simulink model "analiseLongitudinal"  (R2016a)
settings: Solver=ode4  StartTime=0.0  StopTime=60  FixedStep=0.01  RelTol=1e-3
undefined symbols (not defined in the file): aeronave, Ch, Ctheta, CVt, degtorad, Kh, Kq, Ktheta, KVt
libraries: simulink x9, cstblocks x4
settings Model: PauseTimes=20  Creator=IEE  LastModifiedBy=Pegasus
settings DataIOCC: LimitDataPoints=on  SaveFormat=Array
settings DebuggingCC: UnderspecifiedInitializationDetection=Classic  MergeDetectMultiDrivingBlocksExec=none  SolverPrmCheckMsg=warning  StateNameClashWarn=warning
settings HardwareCC: ProdBitPerPointer=32  ProdLargestAtomicFloat=None  ProdIntDivRoundTo=Undefined  ProdEndianess=Unspecified  ProdWordSize=32  ProdHWDeviceType=32-bit Generic
settings ModelReferenceCC: PropagateSignalLabelsOutOfModel=off
settings ConfigComp: CovModelRefEnable=Off

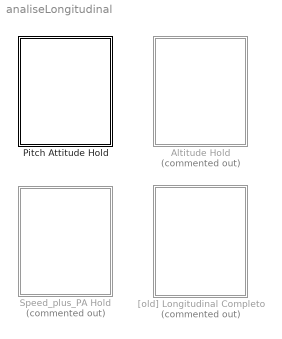
== system analiseLongitudinal ==
  Altitude Hold : Subsystem  Commented=on
  Pitch Attitude Hold : Subsystem
  Speed_plus_PA Hold : Subsystem  Commented=on
  "[old] Longitudinal Completo" : Subsystem  Commented=on

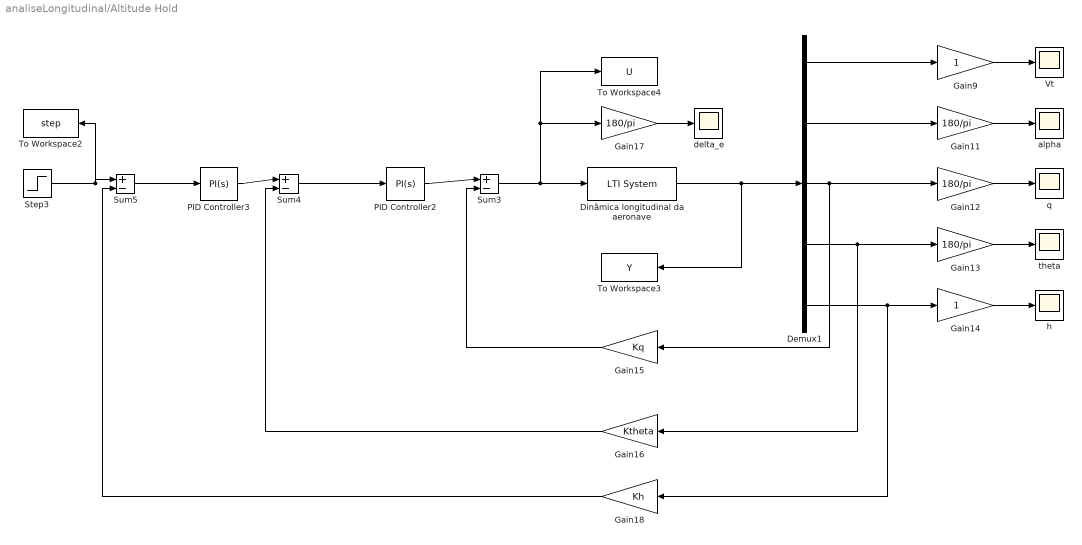
== system analiseLongitudinal/Altitude Hold ==
  Demux1 : Demux  Outputs=5
  Dinâmica longitudinal da aeronave : cstblocks/LTI System  sys=aeronave(:,2)  IC=[]
  Gain{11..13,17} (4 alike) : Gain  Gain=180/pi
  Gain14 : Gain
  Gain15 : Gain  Gain=Kq
  Gain16 : Gain  Gain=Ktheta
  Gain18 : Gain  Gain=Kh
  Gain9 : Gain
  PID Controller2 : simulink/Continuous/PID Controller  Controller=PI  TimeDomain=Continuous-time  SampleTime=-1  IntegratorMethod=Forward Euler  FilterMethod=Forward Euler  Form=Parallel  UseFilter=on  ControllerParametersSource=internal  P=Ctheta.Kp  I=Ctheta.Ki  D=0  N=100  InitialConditionSource=internal  InitialConditionForIntegrator=0  InitialConditionForFilter=0  ExternalReset=none  LimitOutput=off  UpperSaturationLimit=inf  LowerSaturationLimit=-inf  LinearizeAsGain=on  AntiWindupMode=none  Kb=1  TrackingMode=off  Kt=1  PParamMin=[]  PParamMax=[]  IParamMin=[]  IParamMax=[]  DParamMin=[]  DParamMax=[]  NParamMin=[]  NParamMax=[]  KbParamMin=[]  KbParamMax=[]  KtParamMin=[]  KtParamMax=[]  POutMin=[]  POutMax=[]  IOutMin=[]  IOutMax=[]  DOutMin=[]  DOutMax=[]  NOutMin=[]  NOutMax=[]  KbOutMin=[]  KbOutMax=[]  KtOutMin=[]  KtOutMax=[]  IntegratorOutMin=[]  IntegratorOutMax=[]  FilterOutMin=[]  FilterOutMax=[]  SumOutMin=[]  SumOutMax=[]  SumI1OutMin=[]  SumI1OutMax=[]  SumI2OutMin=[]  SumI2OutMax=[]  SumI3OutMin=[]  SumI3OutMax=[]  SumDOutMin=[]  SumDOutMax=[]  SaturationOutMin=[]  SaturationOutMax=[]  IntegratorContinuousStateAttributes=''  IntegratorStateMustResolveToSignalObject=off  IntegratorRTWStateStorageClass=Auto  FilterContinuousStateAttributes=''  FilterStateMustResolveToSignalObject=off  FilterRTWStateStorageClass=Auto  DifferentiatorICPrevScaledInput=0  DifferentiatorOutMin=[]  DifferentiatorOutMax=[]
  PID Controller3 : simulink/Continuous/PID Controller  Controller=PI  TimeDomain=Continuous-time  SampleTime=-1  IntegratorMethod=Forward Euler  FilterMethod=Forward Euler  Form=Parallel  UseFilter=on  ControllerParametersSource=internal  P=Ch.Kp  I=Ch.Ki  D=0  N=100  InitialConditionSource=internal  InitialConditionForIntegrator=0  InitialConditionForFilter=0  ExternalReset=none  LimitOutput=off  UpperSaturationLimit=inf  LowerSaturationLimit=-inf  LinearizeAsGain=on  AntiWindupMode=none  Kb=1  TrackingMode=off  Kt=1  PParamMin=[]  PParamMax=[]  IParamMin=[]  IParamMax=[]  DParamMin=[]  DParamMax=[]  NParamMin=[]  NParamMax=[]  KbParamMin=[]  KbParamMax=[]  KtParamMin=[]  KtParamMax=[]  POutMin=[]  POutMax=[]  IOutMin=[]  IOutMax=[]  DOutMin=[]  DOutMax=[]  NOutMin=[]  NOutMax=[]  KbOutMin=[]  KbOutMax=[]  KtOutMin=[]  KtOutMax=[]  IntegratorOutMin=[]  IntegratorOutMax=[]  FilterOutMin=[]  FilterOutMax=[]  SumOutMin=[]  SumOutMax=[]  SumI1OutMin=[]  SumI1OutMax=[]  SumI2OutMin=[]  SumI2OutMax=[]  SumI3OutMin=[]  SumI3OutMax=[]  SumDOutMin=[]  SumDOutMax=[]  SaturationOutMin=[]  SaturationOutMax=[]  IntegratorContinuousStateAttributes=''  IntegratorStateMustResolveToSignalObject=off  IntegratorRTWStateStorageClass=Auto  FilterContinuousStateAttributes=''  FilterStateMustResolveToSignalObject=off  FilterRTWStateStorageClass=Auto  DifferentiatorICPrevScaledInput=0  DifferentiatorOutMin=[]  DifferentiatorOutMax=[]
  Step3 : Step  Time=20  After=5  SampleTime=0
  Sum3 : Sum  Inputs=|+-
  Sum4 : Sum  Inputs=|+-
  Sum5 : Sum  Inputs=|+-
  To Workspace2 : ToWorkspace  VariableName=step  SaveFormat=Timeseries  SampleTime=-1
  To Workspace3 : ToWorkspace  VariableName=Y  SaveFormat=Timeseries  SampleTime=-1
  To Workspace4 : ToWorkspace  VariableName=U  SaveFormat=Timeseries  SampleTime=-1
  Vt : Scope
  alpha : Scope
  delta_e : Scope
  h : Scope
  q : Scope
  theta : Scope
  wires:
  Demux1/1 -> Gain9/1
  Gain12/1 -> q/1
  Gain14/1 -> h/1
  Gain13/1 -> theta/1
  Demux1/2 -> Gain11/1
  Demux1/3 -> Gain15/1, Gain12/1
  Gain9/1 -> Vt/1
  Gain15/1 -> Sum3/2
  Gain11/1 -> alpha/1
  Gain16/1 -> Sum4/2
  PID Controller2/1 -> Sum3/1
  Gain17/1 -> delta_e/1
  Demux1/4 -> Gain16/1, Gain13/1
  Dinâmica longitudinal da aeronave/1 -> To Workspace3/1, Demux1/1
  Sum3/1 -> To Workspace4/1, Gain17/1, Dinâmica longitudinal da aeronave/1
  Demux1/5 -> Gain18/1, Gain14/1
  Step3/1 -> To Workspace2/1, Sum5/1
  Gain18/1 -> Sum5/2
  Sum5/1 -> PID Controller3/1
  PID Controller3/1 -> Sum4/1
  Sum4/1 -> PID Controller2/1

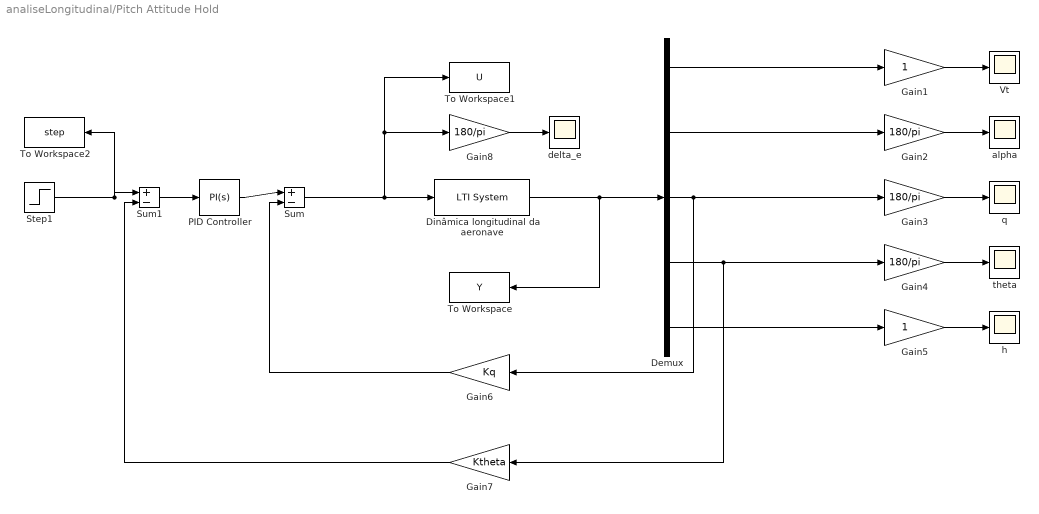
== system analiseLongitudinal/Pitch Attitude Hold ==
  Demux : Demux  Outputs=5
  Dinâmica longitudinal da aeronave : cstblocks/LTI System  sys=aeronave(:,2)  IC=[]
  Gain1 : Gain
  Gain{2..4,8} (4 alike) : Gain  Gain=180/pi
  Gain5 : Gain
  Gain6 : Gain  Gain=Kq
  Gain7 : Gain  Gain=Ktheta
  PID Controller : simulink/Continuous/PID Controller  Controller=PI  TimeDomain=Continuous-time  SampleTime=-1  IntegratorMethod=Forward Euler  FilterMethod=Forward Euler  Form=Parallel  UseFilter=on  ControllerParametersSource=internal  P=Ctheta.Kp  I=Ctheta.Ki  D=0  N=100  InitialConditionSource=internal  InitialConditionForIntegrator=0  InitialConditionForFilter=0  ExternalReset=none  LimitOutput=off  UpperSaturationLimit=inf  LowerSaturationLimit=-inf  LinearizeAsGain=on  AntiWindupMode=none  Kb=1  TrackingMode=off  Kt=1  PParamMin=[]  PParamMax=[]  IParamMin=[]  IParamMax=[]  DParamMin=[]  DParamMax=[]  NParamMin=[]  NParamMax=[]  KbParamMin=[]  KbParamMax=[]  KtParamMin=[]  KtParamMax=[]  POutMin=[]  POutMax=[]  IOutMin=[]  IOutMax=[]  DOutMin=[]  DOutMax=[]  NOutMin=[]  NOutMax=[]  KbOutMin=[]  KbOutMax=[]  KtOutMin=[]  KtOutMax=[]  IntegratorOutMin=[]  IntegratorOutMax=[]  FilterOutMin=[]  FilterOutMax=[]  SumOutMin=[]  SumOutMax=[]  SumI1OutMin=[]  SumI1OutMax=[]  SumI2OutMin=[]  SumI2OutMax=[]  SumI3OutMin=[]  SumI3OutMax=[]  SumDOutMin=[]  SumDOutMax=[]  SaturationOutMin=[]  SaturationOutMax=[]  IntegratorContinuousStateAttributes=''  IntegratorStateMustResolveToSignalObject=off  IntegratorRTWStateStorageClass=Auto  FilterContinuousStateAttributes=''  FilterStateMustResolveToSignalObject=off  FilterRTWStateStorageClass=Auto  DifferentiatorICPrevScaledInput=0  DifferentiatorOutMin=[]  DifferentiatorOutMax=[]
  Step1 : Step  Time=20  After=degtorad(5)  SampleTime=0
  Sum : Sum  Inputs=|+-
  Sum1 : Sum  Inputs=|+-
  To Workspace : ToWorkspace  VariableName=Y  SaveFormat=Timeseries  SampleTime=-1
  To Workspace1 : ToWorkspace  VariableName=U  SaveFormat=Timeseries  SampleTime=-1
  To Workspace2 : ToWorkspace  VariableName=step  SaveFormat=Timeseries  SampleTime=-1
  Vt : Scope
  alpha : Scope
  delta_e : Scope
  h : Scope
  q : Scope
  theta : Scope
  wires:
  Demux/1 -> Gain1/1
  Gain3/1 -> q/1
  Gain5/1 -> h/1
  Demux/5 -> Gain5/1
  Gain4/1 -> theta/1
  Demux/2 -> Gain2/1
  Demux/3 -> Gain6/1, Gain3/1
  Gain1/1 -> Vt/1
  Gain6/1 -> Sum/2
  Gain2/1 -> alpha/1
  Gain7/1 -> Sum1/2
  PID Controller/1 -> Sum/1
  Sum1/1 -> PID Controller/1
  Step1/1 -> To Workspace2/1, Sum1/1
  Gain8/1 -> delta_e/1
  Demux/4 -> Gain7/1, Gain4/1
  Dinâmica longitudinal da aeronave/1 -> To Workspace/1, Demux/1
  Sum/1 -> To Workspace1/1, Gain8/1, Dinâmica longitudinal da aeronave/1

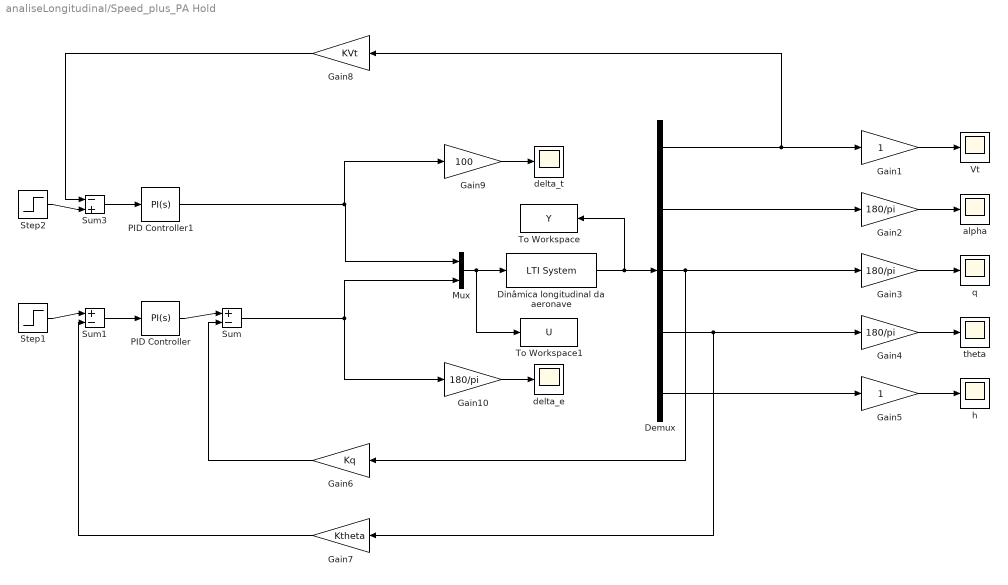
== system analiseLongitudinal/Speed_plus_PA Hold ==
  Demux : Demux  Outputs=5
  Dinâmica longitudinal da aeronave : cstblocks/LTI System  sys=aeronave  IC=[]
  Gain1 : Gain
  Gain{2..4,10} (4 alike) : Gain  Gain=180/pi
  Gain5 : Gain
  Gain6 : Gain  Gain=Kq
  Gain7 : Gain  Gain=Ktheta
  Gain8 : Gain  Gain=KVt
  Gain9 : Gain  Gain=100
  Mux : Mux  Inputs=2
  PID Controller : simulink/Continuous/PID Controller  Controller=PI  TimeDomain=Continuous-time  SampleTime=-1  IntegratorMethod=Forward Euler  FilterMethod=Forward Euler  Form=Parallel  UseFilter=on  ControllerParametersSource=internal  P=Ctheta.Kp  I=Ctheta.Ki  D=0  N=100  InitialConditionSource=internal  InitialConditionForIntegrator=0  InitialConditionForFilter=0  ExternalReset=none  LimitOutput=off  UpperSaturationLimit=inf  LowerSaturationLimit=-inf  LinearizeAsGain=on  AntiWindupMode=none  Kb=1  TrackingMode=off  Kt=1  PParamMin=[]  PParamMax=[]  IParamMin=[]  IParamMax=[]  DParamMin=[]  DParamMax=[]  NParamMin=[]  NParamMax=[]  KbParamMin=[]  KbParamMax=[]  KtParamMin=[]  KtParamMax=[]  POutMin=[]  POutMax=[]  IOutMin=[]  IOutMax=[]  DOutMin=[]  DOutMax=[]  NOutMin=[]  NOutMax=[]  KbOutMin=[]  KbOutMax=[]  KtOutMin=[]  KtOutMax=[]  IntegratorOutMin=[]  IntegratorOutMax=[]  FilterOutMin=[]  FilterOutMax=[]  SumOutMin=[]  SumOutMax=[]  SumI1OutMin=[]  SumI1OutMax=[]  SumI2OutMin=[]  SumI2OutMax=[]  SumI3OutMin=[]  SumI3OutMax=[]  SumDOutMin=[]  SumDOutMax=[]  SaturationOutMin=[]  SaturationOutMax=[]  IntegratorContinuousStateAttributes=''  IntegratorStateMustResolveToSignalObject=off  IntegratorRTWStateStorageClass=Auto  FilterContinuousStateAttributes=''  FilterStateMustResolveToSignalObject=off  FilterRTWStateStorageClass=Auto  DifferentiatorICPrevScaledInput=0  DifferentiatorOutMin=[]  DifferentiatorOutMax=[]
  PID Controller1 : simulink/Continuous/PID Controller  Controller=PI  TimeDomain=Continuous-time  SampleTime=-1  IntegratorMethod=Forward Euler  FilterMethod=Forward Euler  Form=Parallel  UseFilter=on  ControllerParametersSource=internal  P=CVt.Kp  I=CVt.Ki  D=0  N=100  InitialConditionSource=internal  InitialConditionForIntegrator=0  InitialConditionForFilter=0  ExternalReset=none  LimitOutput=off  UpperSaturationLimit=inf  LowerSaturationLimit=-inf  LinearizeAsGain=on  AntiWindupMode=none  Kb=1  TrackingMode=off  Kt=1  PParamMin=[]  PParamMax=[]  IParamMin=[]  IParamMax=[]  DParamMin=[]  DParamMax=[]  NParamMin=[]  NParamMax=[]  KbParamMin=[]  KbParamMax=[]  KtParamMin=[]  KtParamMax=[]  POutMin=[]  POutMax=[]  IOutMin=[]  IOutMax=[]  DOutMin=[]  DOutMax=[]  NOutMin=[]  NOutMax=[]  KbOutMin=[]  KbOutMax=[]  KtOutMin=[]  KtOutMax=[]  IntegratorOutMin=[]  IntegratorOutMax=[]  FilterOutMin=[]  FilterOutMax=[]  SumOutMin=[]  SumOutMax=[]  SumI1OutMin=[]  SumI1OutMax=[]  SumI2OutMin=[]  SumI2OutMax=[]  SumI3OutMin=[]  SumI3OutMax=[]  SumDOutMin=[]  SumDOutMax=[]  SaturationOutMin=[]  SaturationOutMax=[]  IntegratorContinuousStateAttributes=''  IntegratorStateMustResolveToSignalObject=off  IntegratorRTWStateStorageClass=Auto  FilterContinuousStateAttributes=''  FilterStateMustResolveToSignalObject=off  FilterRTWStateStorageClass=Auto  DifferentiatorICPrevScaledInput=0  DifferentiatorOutMin=[]  DifferentiatorOutMax=[]
  Step1 : Step  Time=20  After=degtorad(5)  SampleTime=0
  Step2 : Step  Time=20  After=0  SampleTime=0
  Sum : Sum  Inputs=|+-
  Sum1 : Sum  Inputs=|+-
  Sum3 : Sum  Inputs=-+|
  To Workspace : ToWorkspace  VariableName=Y  SaveFormat=Timeseries  SampleTime=-1
  To Workspace1 : ToWorkspace  VariableName=U  SaveFormat=Timeseries  SampleTime=-1
  Vt : Scope
  alpha : Scope
  delta_e : Scope
  delta_t : Scope
  h : Scope
  q : Scope
  theta : Scope
  wires:
  Demux/1 -> Gain8/1, Gain1/1
  Gain3/1 -> q/1
  Gain5/1 -> h/1
  Demux/5 -> Gain5/1
  Gain4/1 -> theta/1
  Demux/2 -> Gain2/1
  Demux/3 -> Gain6/1, Gain3/1
  Gain1/1 -> Vt/1
  Gain6/1 -> Sum/2
  Gain2/1 -> alpha/1
  Gain7/1 -> Sum1/2
  PID Controller/1 -> Sum/1
  Sum1/1 -> PID Controller/1
  Demux/4 -> Gain7/1, Gain4/1
  Dinâmica longitudinal da aeronave/1 -> Demux/1, To Workspace/1
  Mux/1 -> To Workspace1/1, Dinâmica longitudinal da aeronave/1
  Step2/1 -> Sum3/2
  Sum3/1 -> PID Controller1/1
  Step1/1 -> Sum1/1
  Gain9/1 -> delta_t/1
  Gain10/1 -> delta_e/1
  Gain8/1 -> Sum3/1
  PID Controller1/1 -> Gain9/1, Mux/1
  Sum/1 -> Gain10/1, Mux/2

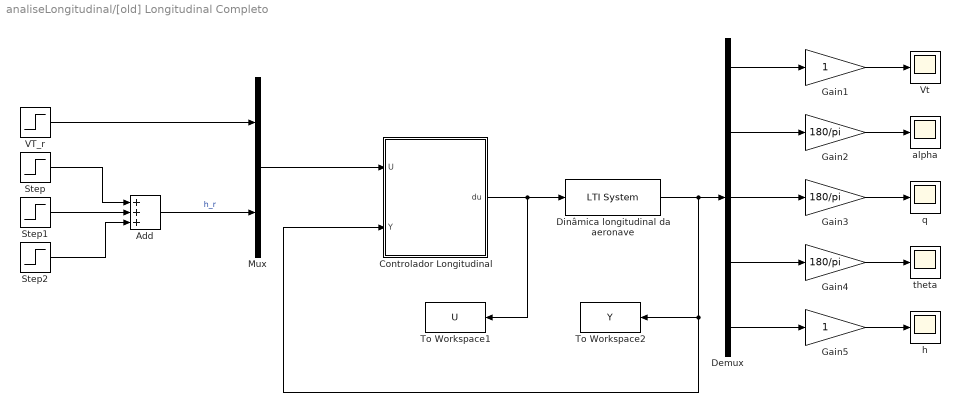
== system analiseLongitudinal/[old] Longitudinal Completo ==
  Add : Sum  Inputs=+++
  Controlador Longitudinal : Subsystem
  Demux : Demux  Outputs=5
  Dinâmica longitudinal da aeronave : cstblocks/LTI System  sys=aeronave  IC=[]
  Gain1 : Gain
  Gain2 : Gain  Gain=180/pi
  Gain3 : Gain  Gain=180/pi
  Gain4 : Gain  Gain=180/pi
  Gain5 : Gain
  Mux : Mux  Inputs=2
  Step : Step  Time=50  After=25  SampleTime=0
  Step1 : Step  Time=150  After=-50  SampleTime=0
  Step2 : Step  Time=250  After=25  SampleTime=0
  To Workspace1 : ToWorkspace  VariableName=U  SaveFormat=Timeseries  SampleTime=-1
  To Workspace2 : ToWorkspace  VariableName=Y  SaveFormat=Timeseries  SampleTime=-1
  VT_r : Step  Time=0  After=0  SampleTime=0
  Vt : Scope
  alpha : Scope
  h : Scope
  q : Scope
  theta : Scope
  wires:
  Demux/1 -> Gain1/1
  Gain3/1 -> q/1
  Gain5/1 -> h/1
  Demux/5 -> Gain5/1
  Gain4/1 -> theta/1
  Demux/2 -> Gain2/1
  Demux/3 -> Gain3/1
  Gain1/1 -> Vt/1
  Gain2/1 -> alpha/1
  Demux/4 -> Gain4/1
  Dinâmica longitudinal da aeronave/1 -> Controlador Longitudinal/2(Y), To Workspace2/1, Demux/1
  Controlador Longitudinal/1(du) -> Dinâmica longitudinal da aeronave/1, To Workspace1/1
  VT_r/1 -> Mux/1
  Step/1 -> Add/1
  Add/1 -> Mux/2  "h_r"
  Step1/1 -> Add/2
  Step2/1 -> Add/3
  Mux/1 -> Controlador Longitudinal/1(U)

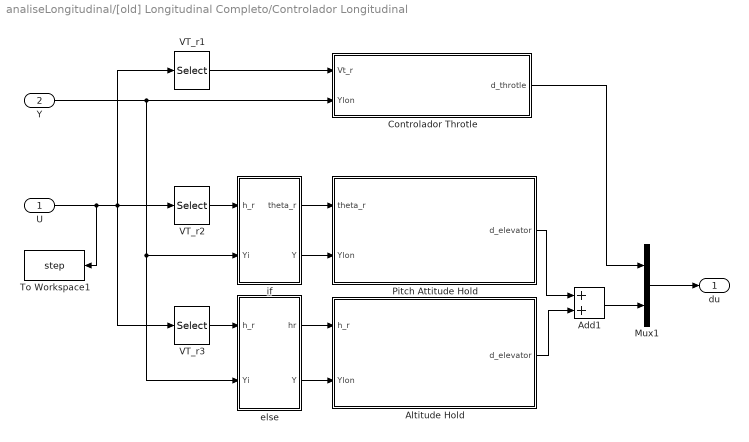
== system analiseLongitudinal/[old] Longitudinal Completo/Controlador Longitudinal ==
  U : Inport
  Y : Inport  Port=2
  Add1 : Sum
  Altitude Hold : Subsystem
  Controlador Throtle : Subsystem
  Mux1 : Mux  Inputs=2
  Pitch Attitude Hold : Subsystem
  To Workspace1 : ToWorkspace  VariableName=step  SaveFormat=Timeseries  SampleTime=-1
  VT_r1 : Selector  InputPortWidth=2  IndexOptions=Index vector (dialog)  Indices=[1]  OutputSizes=1
  VT_r2 : Selector  InputPortWidth=2  IndexOptions=Index vector (dialog)  Indices=[2]  OutputSizes=1
  VT_r3 : Selector  InputPortWidth=2  IndexOptions=Index vector (dialog)  Indices=[2]  OutputSizes=1
  else : Subsystem
  if : Subsystem
  du : Outport
  wires:
  Pitch Attitude Hold/1(d_elevator) -> Add1/1
  Controlador Throtle/1(d_throtle) -> Mux1/1
  Altitude Hold/1(d_elevator) -> Add1/2
  Mux1/1 -> du/1
  if/2(Y) -> Pitch Attitude Hold/2(Ylon)
  Add1/1 -> Mux1/2
  if/1(theta_r) -> Pitch Attitude Hold/1(theta_r)
  else/2(Y) -> Altitude Hold/2(Ylon)
  else/1(hr) -> Altitude Hold/1(h_r)
  VT_r3/1 -> else/1(h_r)
  VT_r2/1 -> if/1(h_r)
  VT_r1/1 -> Controlador Throtle/1(Vt_r)
  Y/1 -> if/2(Yi), else/2(Yi), Controlador Throtle/2(Ylon)
  U/1 -> To Workspace1/1, VT_r1/1, VT_r3/1, VT_r2/1

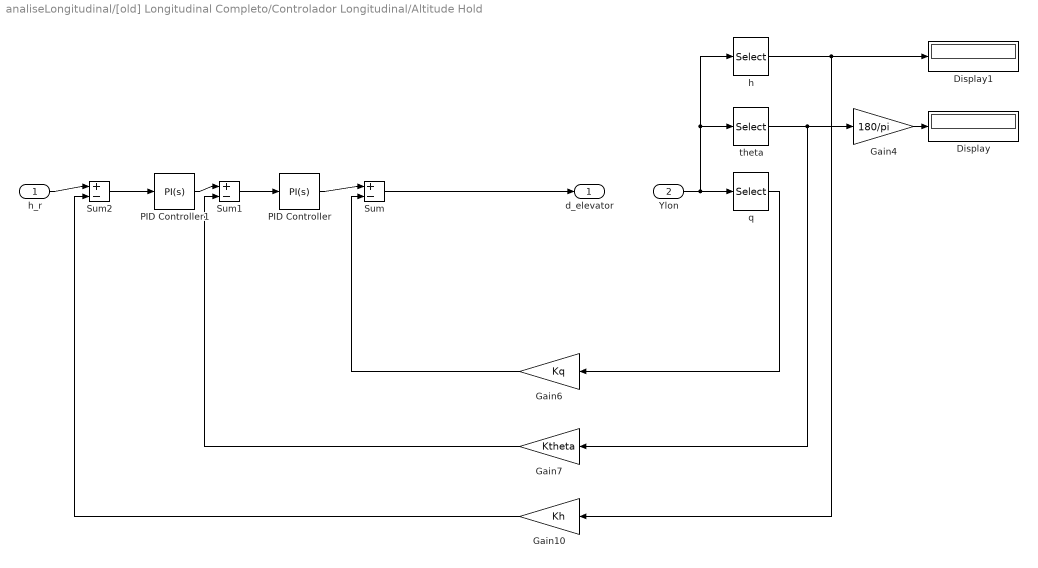
== system analiseLongitudinal/[old] Longitudinal Completo/Controlador Longitudinal/Altitude Hold ==
  h_r : Inport
  Ylon : Inport  Port=2
  Display : Display
  Display1 : Display
  Gain10 : Gain  Gain=Kh
  Gain4 : Gain  Gain=180/pi
  Gain6 : Gain  Gain=Kq
  Gain7 : Gain  Gain=Ktheta
  PID Controller : simulink/Continuous/PID Controller  Controller=PI  TimeDomain=Continuous-time  SampleTime=-1  IntegratorMethod=Forward Euler  FilterMethod=Forward Euler  Form=Parallel  UseFilter=on  ControllerParametersSource=internal  P=Ctheta.Kp  I=Ctheta.Ki  D=0  N=100  InitialConditionSource=internal  InitialConditionForIntegrator=0  InitialConditionForFilter=0  ExternalReset=none  LimitOutput=off  UpperSaturationLimit=inf  LowerSaturationLimit=-inf  LinearizeAsGain=on  AntiWindupMode=none  Kb=1  TrackingMode=off  Kt=1  PParamMin=[]  PParamMax=[]  IParamMin=[]  IParamMax=[]  DParamMin=[]  DParamMax=[]  NParamMin=[]  NParamMax=[]  KbParamMin=[]  KbParamMax=[]  KtParamMin=[]  KtParamMax=[]  POutMin=[]  POutMax=[]  IOutMin=[]  IOutMax=[]  DOutMin=[]  DOutMax=[]  NOutMin=[]  NOutMax=[]  KbOutMin=[]  KbOutMax=[]  KtOutMin=[]  KtOutMax=[]  IntegratorOutMin=[]  IntegratorOutMax=[]  FilterOutMin=[]  FilterOutMax=[]  SumOutMin=[]  SumOutMax=[]  SumI1OutMin=[]  SumI1OutMax=[]  SumI2OutMin=[]  SumI2OutMax=[]  SumI3OutMin=[]  SumI3OutMax=[]  SumDOutMin=[]  SumDOutMax=[]  SaturationOutMin=[]  SaturationOutMax=[]  IntegratorContinuousStateAttributes=''  IntegratorStateMustResolveToSignalObject=off  IntegratorRTWStateStorageClass=Auto  FilterContinuousStateAttributes=''  FilterStateMustResolveToSignalObject=off  FilterRTWStateStorageClass=Auto  DifferentiatorICPrevScaledInput=0  DifferentiatorOutMin=[]  DifferentiatorOutMax=[]
  PID Controller1 : simulink/Continuous/PID Controller  Controller=PI  TimeDomain=Continuous-time  SampleTime=-1  IntegratorMethod=Forward Euler  FilterMethod=Forward Euler  Form=Parallel  UseFilter=on  ControllerParametersSource=internal  P=Ch.Kp  I=Ch.Ki  D=0  N=100  InitialConditionSource=internal  InitialConditionForIntegrator=0  InitialConditionForFilter=0  ExternalReset=none  LimitOutput=off  UpperSaturationLimit=inf  LowerSaturationLimit=-inf  LinearizeAsGain=on  AntiWindupMode=none  Kb=1  TrackingMode=off  Kt=1  PParamMin=[]  PParamMax=[]  IParamMin=[]  IParamMax=[]  DParamMin=[]  DParamMax=[]  NParamMin=[]  NParamMax=[]  KbParamMin=[]  KbParamMax=[]  KtParamMin=[]  KtParamMax=[]  POutMin=[]  POutMax=[]  IOutMin=[]  IOutMax=[]  DOutMin=[]  DOutMax=[]  NOutMin=[]  NOutMax=[]  KbOutMin=[]  KbOutMax=[]  KtOutMin=[]  KtOutMax=[]  IntegratorOutMin=[]  IntegratorOutMax=[]  FilterOutMin=[]  FilterOutMax=[]  SumOutMin=[]  SumOutMax=[]  SumI1OutMin=[]  SumI1OutMax=[]  SumI2OutMin=[]  SumI2OutMax=[]  SumI3OutMin=[]  SumI3OutMax=[]  SumDOutMin=[]  SumDOutMax=[]  SaturationOutMin=[]  SaturationOutMax=[]  IntegratorContinuousStateAttributes=''  IntegratorStateMustResolveToSignalObject=off  IntegratorRTWStateStorageClass=Auto  FilterContinuousStateAttributes=''  FilterStateMustResolveToSignalObject=off  FilterRTWStateStorageClass=Auto  DifferentiatorICPrevScaledInput=0  DifferentiatorOutMin=[]  DifferentiatorOutMax=[]
  Sum : Sum  Inputs=|+-
  Sum1 : Sum  Inputs=|+-
  Sum2 : Sum  Inputs=|+-
  h : Selector  InputPortWidth=5  IndexOptions=Index vector (dialog)  Indices=[5]  OutputSizes=1
  q : Selector  InputPortWidth=5  IndexOptions=Index vector (dialog)  Indices=[3]  OutputSizes=1
  theta : Selector  InputPortWidth=5  IndexOptions=Index vector (dialog)  Indices=[4]  OutputSizes=1
  d_elevator : Outport
  wires:
  Gain6/1 -> Sum/2
  Gain7/1 -> Sum1/2
  PID Controller/1 -> Sum/1
  Sum1/1 -> PID Controller/1
  PID Controller1/1 -> Sum1/1
  Gain10/1 -> Sum2/2
  Sum2/1 -> PID Controller1/1
  theta/1 -> Gain7/1, Gain4/1
  q/1 -> Gain6/1
  Ylon/1 -> theta/1, h/1, q/1
  h/1 -> Display1/1, Gain10/1
  Sum/1 -> d_elevator/1
  h_r/1 -> Sum2/1
  Gain4/1 -> Display/1

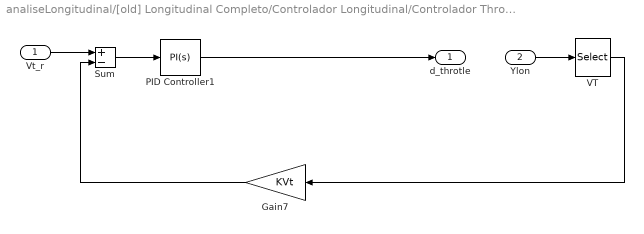
== system analiseLongitudinal/[old] Longitudinal Completo/Controlador Longitudinal/Controlador Throtle ==
  Vt_r : Inport
  Ylon : Inport  Port=2
  Gain7 : Gain  Gain=KVt
  PID Controller1 : simulink/Continuous/PID Controller  Controller=PI  TimeDomain=Continuous-time  SampleTime=-1  IntegratorMethod=Forward Euler  FilterMethod=Forward Euler  Form=Parallel  UseFilter=on  ControllerParametersSource=internal  P=CVt.Kp  I=CVt.Ki  D=0  N=100  InitialConditionSource=internal  InitialConditionForIntegrator=0  InitialConditionForFilter=0  ExternalReset=none  LimitOutput=off  UpperSaturationLimit=inf  LowerSaturationLimit=-inf  LinearizeAsGain=on  AntiWindupMode=none  Kb=1  TrackingMode=off  Kt=1  PParamMin=[]  PParamMax=[]  IParamMin=[]  IParamMax=[]  DParamMin=[]  DParamMax=[]  NParamMin=[]  NParamMax=[]  KbParamMin=[]  KbParamMax=[]  KtParamMin=[]  KtParamMax=[]  POutMin=[]  POutMax=[]  IOutMin=[]  IOutMax=[]  DOutMin=[]  DOutMax=[]  NOutMin=[]  NOutMax=[]  KbOutMin=[]  KbOutMax=[]  KtOutMin=[]  KtOutMax=[]  IntegratorOutMin=[]  IntegratorOutMax=[]  FilterOutMin=[]  FilterOutMax=[]  SumOutMin=[]  SumOutMax=[]  SumI1OutMin=[]  SumI1OutMax=[]  SumI2OutMin=[]  SumI2OutMax=[]  SumI3OutMin=[]  SumI3OutMax=[]  SumDOutMin=[]  SumDOutMax=[]  SaturationOutMin=[]  SaturationOutMax=[]  IntegratorContinuousStateAttributes=''  IntegratorStateMustResolveToSignalObject=off  IntegratorRTWStateStorageClass=Auto  FilterContinuousStateAttributes=''  FilterStateMustResolveToSignalObject=off  FilterRTWStateStorageClass=Auto  DifferentiatorICPrevScaledInput=0  DifferentiatorOutMin=[]  DifferentiatorOutMax=[]
  Sum : Sum  Inputs=+-
  VT : Selector  InputPortWidth=5  IndexOptions=Index vector (dialog)  Indices=1  OutputSizes=1
  d_throtle : Outport
  wires:
  Sum/1 -> PID Controller1/1
  Vt_r/1 -> Sum/1
  Ylon/1 -> VT/1
  VT/1 -> Gain7/1
  Gain7/1 -> Sum/2
  PID Controller1/1 -> d_throtle/1

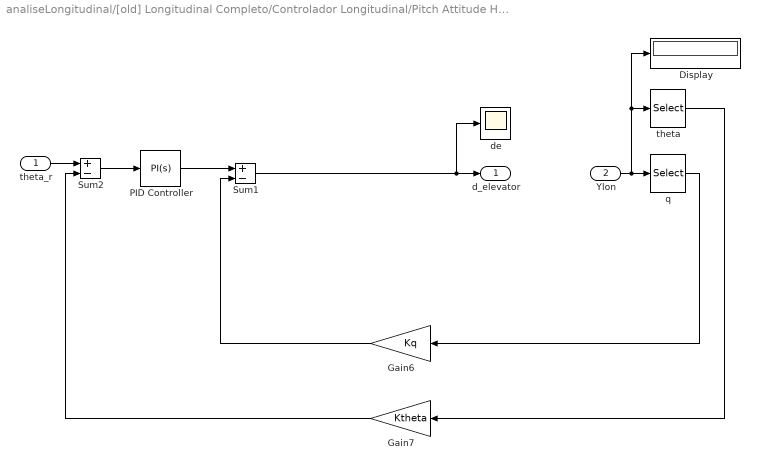
== system analiseLongitudinal/[old] Longitudinal Completo/Controlador Longitudinal/Pitch Attitude Hold ==
  theta_r : Inport
  Ylon : Inport  Port=2
  Display : Display
  Gain6 : Gain  Gain=Kq
  Gain7 : Gain  Gain=Ktheta
  PID Controller : simulink/Continuous/PID Controller  Controller=PI  TimeDomain=Continuous-time  SampleTime=-1  IntegratorMethod=Forward Euler  FilterMethod=Forward Euler  Form=Parallel  UseFilter=on  ControllerParametersSource=internal  P=Ctheta.Kp  I=Ctheta.Ki  D=0  N=100  InitialConditionSource=internal  InitialConditionForIntegrator=0  InitialConditionForFilter=0  ExternalReset=none  LimitOutput=off  UpperSaturationLimit=inf  LowerSaturationLimit=-inf  LinearizeAsGain=on  AntiWindupMode=none  Kb=1  TrackingMode=off  Kt=1  PParamMin=[]  PParamMax=[]  IParamMin=[]  IParamMax=[]  DParamMin=[]  DParamMax=[]  NParamMin=[]  NParamMax=[]  KbParamMin=[]  KbParamMax=[]  KtParamMin=[]  KtParamMax=[]  POutMin=[]  POutMax=[]  IOutMin=[]  IOutMax=[]  DOutMin=[]  DOutMax=[]  NOutMin=[]  NOutMax=[]  KbOutMin=[]  KbOutMax=[]  KtOutMin=[]  KtOutMax=[]  IntegratorOutMin=[]  IntegratorOutMax=[]  FilterOutMin=[]  FilterOutMax=[]  SumOutMin=[]  SumOutMax=[]  SumI1OutMin=[]  SumI1OutMax=[]  SumI2OutMin=[]  SumI2OutMax=[]  SumI3OutMin=[]  SumI3OutMax=[]  SumDOutMin=[]  SumDOutMax=[]  SaturationOutMin=[]  SaturationOutMax=[]  IntegratorContinuousStateAttributes=''  IntegratorStateMustResolveToSignalObject=off  IntegratorRTWStateStorageClass=Auto  FilterContinuousStateAttributes=''  FilterStateMustResolveToSignalObject=off  FilterRTWStateStorageClass=Auto  DifferentiatorICPrevScaledInput=0  DifferentiatorOutMin=[]  DifferentiatorOutMax=[]
  Sum1 : Sum  Inputs=+-
  Sum2 : Sum  Inputs=+-
  de : Scope
  q : Selector  InputPortWidth=5  IndexOptions=Index vector (dialog)  Indices=[3]  OutputSizes=1
  theta : Selector  InputPortWidth=5  IndexOptions=Index vector (dialog)  Indices=[4]  OutputSizes=1
  d_elevator : Outport
  wires:
  theta/1 -> Gain7/1
  q/1 -> Gain6/1
  Gain6/1 -> Sum1/2
  Gain7/1 -> Sum2/2
  PID Controller/1 -> Sum1/1
  Sum2/1 -> PID Controller/1
  Ylon/1 -> Display/1, theta/1, q/1
  Sum1/1 -> de/1, d_elevator/1
  theta_r/1 -> Sum2/1

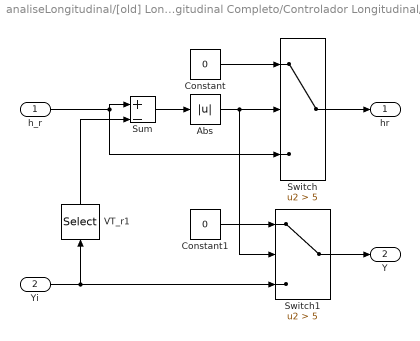
== system analiseLongitudinal/[old] Longitudinal Completo/Controlador Longitudinal/else ==
  h_r : Inport
  Yi : Inport  Port=2
  Abs : Abs
  Constant : Constant  Value=0
  Constant1 : Constant  Value=0
  Sum : Sum  Inputs=|+-
  Switch : Switch  Criteria=u2 > Threshold  Threshold=5
  Switch1 : Switch  Criteria=u2 > Threshold  Threshold=5
  VT_r1 : Selector  InputPortWidth=5  IndexOptions=Index vector (dialog)  Indices=[5]  OutputSizes=1
  hr : Outport
  Y : Outport  Port=2
  wires:
  Abs/1 -> Switch1/2, Switch/2
  Yi/1 -> Switch1/3, VT_r1/1
  Switch/1 -> hr/1
  Sum/1 -> Abs/1
  Switch1/1 -> Y/1
  Constant/1 -> Switch/1
  Constant1/1 -> Switch1/1
  h_r/1 -> Sum/1, Switch/3
  VT_r1/1 -> Sum/2

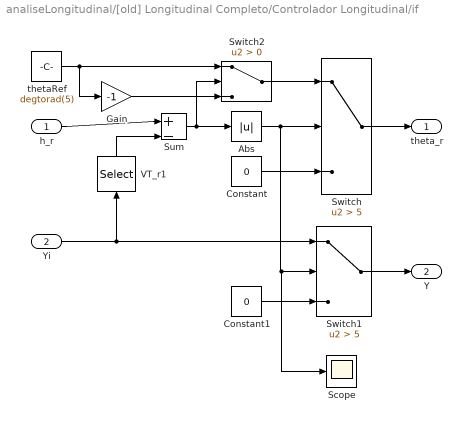
== system analiseLongitudinal/[old] Longitudinal Completo/Controlador Longitudinal/if ==
  h_r : Inport
  Yi : Inport  Port=2
  Abs : Abs
  Constant : Constant  Value=0
  Constant1 : Constant  Value=0
  Gain : Gain  Gain=-1
  Scope : Scope
  Sum : Sum  Inputs=|+-
  Switch : Switch  Criteria=u2 > Threshold  Threshold=5
  Switch1 : Switch  Criteria=u2 > Threshold  Threshold=5
  Switch2 : Switch  Criteria=u2 > Threshold
  VT_r1 : Selector  InputPortWidth=5  IndexOptions=Index vector (dialog)  Indices=[5]  OutputSizes=1
  thetaRef : Constant  Value=degtorad(5)
  theta_r : Outport
  Y : Outport  Port=2
  wires:
  Abs/1 -> Scope/1, Switch1/2, Switch/2
  Switch/1 -> theta_r/1
  h_r/1 -> Sum/1
  Switch1/1 -> Y/1
  Constant/1 -> Switch/3
  Yi/1 -> VT_r1/1, Switch1/1
  Constant1/1 -> Switch1/3
  Gain/1 -> Switch2/3
  thetaRef/1 -> Gain/1, Switch2/1
  Switch2/1 -> Switch/1
  VT_r1/1 -> Sum/2
  Sum/1 -> Switch2/2, Abs/1
